simulink model "task2"  (R2012b)
settings: Solver=ode45  StartTime=0.0  StopTime=10.0  RelTol=1e-3
settings Model: Creator=student-at  LastModifiedBy=student-at

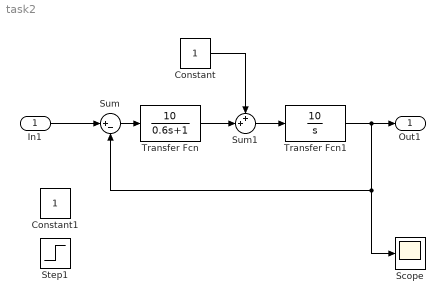
== system task2 ==
  In1 : Inport
  Constant : Constant
  Constant1 : Constant
  Scope : Scope
  Step1 : Step  SampleTime=0
  Sum : Sum  Inputs=|+-
  Sum1 : Sum  Inputs=++|
  Transfer Fcn : TransferFcn  Numerator=[10]  Denominator=[0.6 1]
  Transfer Fcn1 : TransferFcn  Numerator=[10]  Denominator=[1 0]
  Out1 : Outport
  wires:
  Constant/1 -> Sum1/1
  Sum/1 -> Transfer Fcn/1
  Transfer Fcn/1 -> Sum1/2
  Sum1/1 -> Transfer Fcn1/1
  Transfer Fcn1/1 -> Out1/1, Sum/2, Scope/1
  In1/1 -> Sum/1
